simulink model "Exp6_19EE10009_SinglrPhaseInverter"  (R2021a)
settings: Solver=VariableStepAuto  StartTime=0.0  StopTime=10.0  RelTol=1e-3
libraries: spsMosfetLib x4, simulink x2, spsCurrentMeasurementLib x1, spsDCVoltageSourceLib x1, spsSeriesRLCBranchLib x1, spsVoltageMeasurementLib x1, spspowerguiLib x1
settings Model: Creator=ARUNDHUTI  LastModifiedBy=ARUNDHUTI

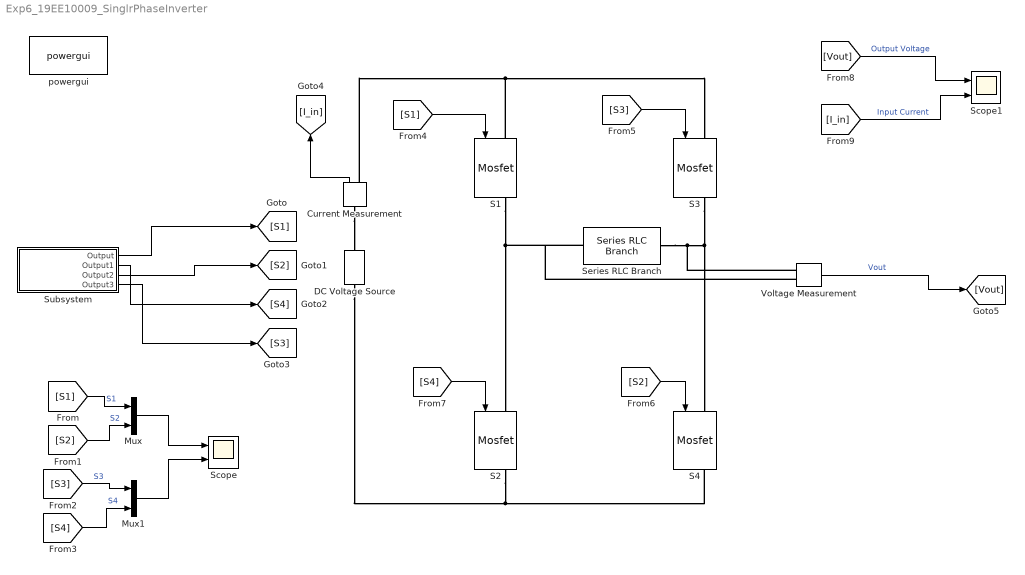
== system Exp6_19EE10009_SinglrPhaseInverter ==
  Current Measurement : spsCurrentMeasurementLib/Current Measurement  PhasorSimulation=off  OutputType=Complex  PSBequivalent=0
  DC Voltage Source : spsDCVoltageSourceLib/DC Voltage Source  Amplitude=400  Measurements=None
  Mux : Mux  Inputs=2
  Mux1 : Mux  Inputs=2
  S{1..4} (4 alike) : spsMosfetLib/Mosfet  Ron=2e-3  Lon=0  Rd=1e-3  Vfd=0.7  IC=0  Rs=1e12  Cs=1e-12  Measurements=on
  Scope : Scope  NumInputPorts=2
  Scope1 : Scope  NumInputPorts=2
  Series RLC Branch : spsSeriesRLCBranchLib/Series RLC Branch  LConnTagsString=__new0  RConnTagsString=__new0  BranchType=R  Resistance=40  Inductance=1e-3  SetiL0=off  InitialCurrent=0  Capacitance=1e-6  Setx0=off  InitialVoltage=0  Measurements=None
  Subsystem : Subsystem
  Voltage Measurement : spsVoltageMeasurementLib/Voltage Measurement  PhasorSimulation=off  OutputType=Complex  PSBequivalent=0
  powergui : spspowerguiLib/powergui  Priority=1  SimulationMode=Discrete  SampleTime=1e-7  frequency=60  Iterations=50  frequencyindice=0  Pbase=100e6  ErrMax=1e-4  UnitsV=kV  UnitsW=MW  buscounter=0  FunctionMessages=off  echomessages=off  EnableUseOfTLC=off  CurrentSourceSwitches=off  DisableSnubberDevices=off  DisableRonSwitches=off  DisableVfSwitches=off  DisplayEquations=off  AutomaticDiscreteSolvers=off  SolverType=Tustin/Backward Euler (TBE)  Interpol=off  ExternalGateDelay=off  methode=off  Ts=100  x0status=blocks  SPID=on  SwTol=0  HookPort=off  NonlinearTolerance=1e-4  nMaxIteration=100  ContinueOnMaxIteration=off  RestoreLinks=warning  ResistiveCurrentMeasurement=off  Frange=[0:2:500]  Ylog=off  Xlog=on  ShowGrid=off  save=off  variable=ZData  structure=0  ZoomFFT=off  StartTime=0.0  cycles=1  DisplayStyle=1  fundamental=60  FreqAxis=off  MaxFrequency=1000  frequencyindicesteady=1  RmsSteady=1  display=off
  wires:
  Mux1/1 -> Scope/2
  [S1] -> Mux/1  "S1"
  [I_in] -> Scope1/2  "Input Current"
  Current Measurement/1 -> [I_in]
  Subsystem/4(Output3) -> [S3]
  [S3] -> Mux1/1  "S3"
  [Vout] -> Scope1/1  "Output Voltage"
  Voltage Measurement/1 -> [Vout]  "Vout"
  [S4] -> S2/1
  [S2] -> S4/1
  [S1] -> S1/1
  [S2] -> Mux/2  "S2"
  Subsystem/2(Output1) -> [S4]
  Subsystem/1(Output) -> [S1]
  [S3] -> S3/1
  Subsystem/3(Output2) -> [S2]
  Mux/1 -> Scope/1
  [S4] -> Mux1/2  "S4"
  connections:
  Current Measurement/RConn1 -- S3/LConn1 -- S1/LConn1
  DC Voltage Source/LConn1 -- S4/RConn1 -- S2/RConn1
  Voltage Measurement/LConn2 -- Series RLC Branch/RConn1 -- S4/LConn1 -- S3/RConn1
  S1/RConn1 -- Series RLC Branch/LConn1 -- Voltage Measurement/LConn1 -- S2/LConn1
  Current Measurement/LConn1 -- DC Voltage Source/RConn1

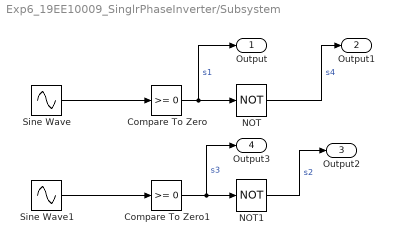
== system Exp6_19EE10009_SinglrPhaseInverter/Subsystem ==
  Compare To Zero : simulink/Logic and Bit Operations/Compare To Zero  relop=>=  OutDataTypeStr=boolean
  Compare To Zero1 : simulink/Logic and Bit Operations/Compare To Zero  relop=>=  OutDataTypeStr=boolean
  NOT : Logic  Operator=NOT  IconShape=distinctive  AllPortsSameDT=off  OutDataTypeStr=boolean
  NOT1 : Logic  Operator=NOT  IconShape=distinctive  AllPortsSameDT=off  OutDataTypeStr=boolean
  Sine Wave : Sin  Frequency=2*pi*50  SampleTime=0
  Sine Wave1 : Sin  Frequency=2*pi*50  Phase=pi  SampleTime=0
  Output : Outport
  Output1 : Outport  Port=2
  Output2 : Outport  Port=3
  Output3 : Outport  Port=4
  wires:
  Sine Wave/1 -> Compare To Zero/1
  Compare To Zero1/1 -> Output3/1, NOT1/1  "s3"
  Sine Wave1/1 -> Compare To Zero1/1
  NOT1/1 -> Output2/1  "s2"
  NOT/1 -> Output1/1  "s4"
  Compare To Zero/1 -> Output/1, NOT/1  "s1"
